simulink model "TestSpace"  (R2016b)
settings: Solver=FixedStepAuto  StartTime=0.0  StopTime=10.0  RelTol=1e-3
settings Model: Creator=NEATdemo  LastModifiedBy=NEATdemo

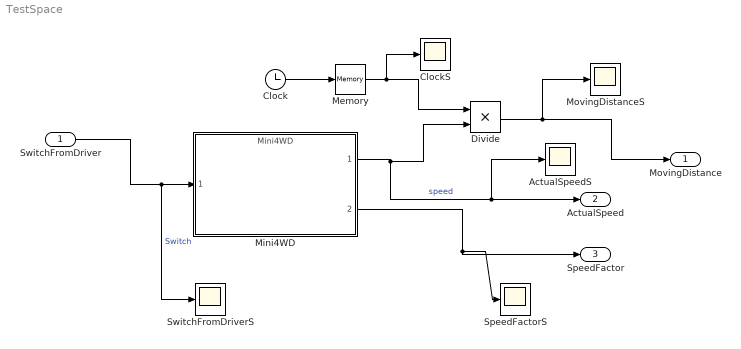
== system TestSpace ==
  SwitchFromDriver : Inport
      settings: AttributesFormatString=Switch
  ActualSpeedS : Scope
  Clock : Clock
  ClockS : Scope
  Divide : Product  Inputs=**
  Memory : Memory
  Mini4WD : ModelReference  ModelNameDialog=Mini4WD  SimulationMode=Normal  ModelReferenceVersion=1.13
  MovingDistanceS : Scope
  SpeedFactorS : Scope
  SwitchFromDriverS : Scope
  MovingDistance : Outport
      settings: AttributesFormatString=Distance
  ActualSpeed : Outport  Port=2
      settings: AttributesFormatString=speed
  SpeedFactor : Outport  Port=3
      settings: AttributesFormatString=SomethingFactor
  wires:
  Mini4WD/1 -> Divide/2, ActualSpeedS/1, ActualSpeed/1  "speed"
  SwitchFromDriver/1 -> SwitchFromDriverS/1, Mini4WD/1  "Switch"
  Mini4WD/2 -> SpeedFactorS/1, SpeedFactor/1
  Clock/1 -> Memory/1
  Memory/1 -> ClockS/1, Divide/1
  Divide/1 -> MovingDistanceS/1, MovingDistance/1
